simulink model "f18full_DUtrim"  (R2015a)
settings: Solver=ode45  StartTime=0.0  StopTime=10.0  RelTol=1e-3
values from neighbouring files (symbols this model uses):
  b = 37.4    [Trim_stab_f18fullDU_a.m]    (also in Trim_stab_f18fullDU_aEDIT.m)
  c = 11.52    [Trim_stab_f18fullDU_a.m]    (also in Trim_stab_f18fullDU_aEDIT.m)
  g = 32.2    [Trim_stab_f18fullDU_a.m]    (also in Trim_stab_f18fullDU_aEDIT.m)
  Ixx = 23000    [Trim_stab_f18fullDU_a.m]    (also in Trim_stab_f18fullDU_aEDIT.m)
  Ixz = - 2971    (= -2971)    [Trim_stab_f18fullDU_a.m]    (also in Trim_stab_f18fullDU_aEDIT.m)
  Iyy = 151293    [Trim_stab_f18fullDU_a.m]    (also in Trim_stab_f18fullDU_aEDIT.m)
  Izz = 169945    [Trim_stab_f18fullDU_a.m]    (also in Trim_stab_f18fullDU_aEDIT.m)
  m = 1034.5    [Trim_stab_f18fullDU_a.m]    (also in Trim_stab_f18fullDU_aEDIT.m)
  rho = 1.0660e-003    (= 0.001066)    [Trim_stab_f18fullDU_a.m]    (also in Trim_stab_f18fullDU_aEDIT.m)
  S = 400    [Trim_stab_f18fullDU_a.m]    (also in Trim_stab_f18fullDU_aEDIT.m)
  x = x_init    [Trim_stab_f18fullDU_a.m]    (also in Trim_stab_f18fullDU_aEDIT.m)
undefined symbols (not defined in the file or in its folder): CD0, CDalpha0, CDalpha1, CDalpha2, CDalpha3, CDalpha4, CDdeltastab0, CDdeltastab1, CDdeltastab2, CDdeltastab3, CLalpha0, CLalpha1, CLalpha2, CLalpha3, CLdeltastab0, CLdeltastab1, CLdeltastab2, CLdeltastab3, CMalpha0, CMalpha1, CMalpha2, CMdeltastab0, CMdeltastab1, CMdeltastab2, CMq0, CMq1, CMq2, CMq3, Cnbeta0, Cnbeta1, Cnbeta2, Cndeltaail0, Cndeltaail1, Cndeltaail2, Cndeltaail3, Cndeltarud0, Cndeltarud1, Cndeltarud2, Cndeltarud3, Cndeltarud4, Cnp0, Cnp1, Cnr0, Cnr1, CYbeta0, CYbeta1, CYbeta2, CYdeltaail0, CYdeltaail1, CYdeltaail2, CYdeltaail3, CYdeltarud0, CYdeltarud1, CYdeltarud2, CYdeltarud3
settings Model: Creator=BC  LastModifiedBy=BC
settings DataIOCC: SignalLoggingSaveFormat=ModelDataLogs
settings OptimizationCC: ExpressionDepthLimit=2147483647
settings DebuggingCC: UnderspecifiedInitializationDetection=Classic  MergeDetectMultiDrivingBlocksExec=none  SolverPrmCheckMsg=warning  FcnCallInpInsideContextMsg=EnableAllAsWarning  StateNameClashWarn=warning
settings GRTTargetCC: CombineOutputUpdateFcns=off  GRTInterface=on

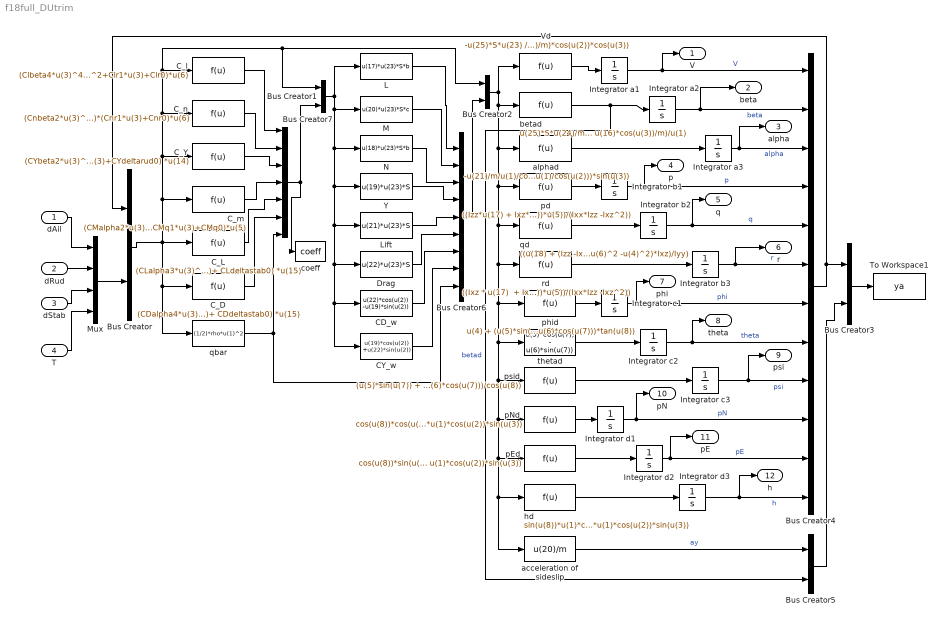
== system f18full_DUtrim ==
  dAil : Inport
  dRud : Inport  Port=2
  dStab : Inport  Port=3
  T : Inport  Port=4
  Bus Creator{,1..3,5} (5 alike) : BusCreator  Inputs=2
  Bus Creator4 : BusCreator  Inputs=12
  Bus Creator6 : BusCreator  Inputs=9
  Bus Creator7 : BusCreator  Inputs=7
  CD_w : Fcn  Expr=u(22)*cos(u(2)) -u(19)*sin(u(2))
  CY_w : Fcn  Expr=u(19)*cos(u(2)) +u(22)*sin(u(2))
  C_D : Fcn  Expr=(CDalpha4*u(3)^4+CDalpha3*u(3)^3+CDalpha2*u(3)^2+CDalpha1*u(3)+CDalpha0)*cos(u(2))+CD0 +(CDdeltastab3*u(3)^3+ CDdeltastab2*u(3)^2+ CDdeltastab1*u(3)+ CDdeltastab0) *u(15)
  C_L : Fcn  Expr=(CLalpha3*u(3)^3+CLalpha2*u(3)^2+CLalpha1*u(3)+CLalpha0)*cos(2*u(2)/3)+(CLdeltastab3*u(3)^3+ CLdeltastab2*u(3)^2+ CLdeltastab1*u(3)+ CLdeltastab0) *u(15)
  C_Y : Fcn  Expr=(CYbeta2*u(3)^2+CYbeta1*u(3)+CYbeta0)*u(2)+(CYdeltaail3*u(3)^3+CYdeltaail2*u(3)^2+CYdeltaail1*u(3)+CYdeltaail0)*u(13)+(CYdeltarud3*u(3)^3+CYdeltarud2*u(3)^2+CYdeltarud1*u(3)+CYdeltarud0) *u(14)
  C_l : Fcn  Expr=(Clbeta4*u(3)^4+Clbeta3*u(3)^3+Clbeta2*u(3)^2+Clbeta1*u(3)+Clbeta0)*u(2)+(Cldeltaail3*u(3)^3+Cldeltaail2*u(3)^2+Cldeltaail1*u(3)+Cldeltaail0)*u(13)+(Cldeltarud3*u(3)^3+Cldeltarud2*u(3)^2+Cldeltarud1*u(3)+Cldeltarud0)*u(14)+(b/(2*u(1)))*(Clp1*u(3)+Clp0)*u(4)+(b/(2*u(1)))*(Clr2*u(3)^2+Clr1*u(3)+Clr0)*u(6)
  C_m : Fcn  Expr=(CMalpha2*u(3)^2+CMalpha1*u(3)+CMalpha0)+(CMdeltastab2*u(3)^2+CMdeltastab1*u(3)+CMdeltastab0)*u(15)+(c/(2*u(1)))*(CMq3*u(3)^3+CMq2*u(3)^2+CMq1*u(3)+CMq0)*u(5)
  C_n : Fcn  Expr=(Cnbeta2*u(3)^2+Cnbeta1*u(3)+Cnbeta0)*u(2)+(Cndeltarud4*u(3)^4+Cndeltarud3*u(3)^3+Cndeltarud2*u(3)^2+Cndeltarud1*u(3)+Cndeltarud0)*u(14)+(Cndeltaail3*u(3)^3+Cndeltaail2*u(3)^2+Cndeltaail1*u(3)+Cndeltaail0)*u(13)+(b/(2*u(1)))*(Cnp1*u(3)+Cnp0)*u(4)+(b/(2*u(1)))*(Cnr1*u(3)+Cnr0)*u(6)
  Drag : Fcn  Expr=u(22)*u(23)*S
  Integrator a1 : Integrator  InitialCondition=x(1)
  Integrator a2 : Integrator  InitialCondition=x(2)
  Integrator a3 : Integrator  InitialCondition=x(3)
  Integrator b1 : Integrator  InitialCondition=x(4)
  Integrator b2 : Integrator  InitialCondition=x(5)
  Integrator b3 : Integrator  InitialCondition=x(6)
  Integrator c1 : Integrator  InitialCondition=x(7)
  Integrator c2 : Integrator  InitialCondition=x(8)
  Integrator c3 : Integrator  InitialCondition=x(9)
  Integrator d1 : Integrator  InitialCondition=x(10)
  Integrator d2 : Integrator  InitialCondition=x(11)
  Integrator d3 : Integrator  InitialCondition=x(12)
  L : Fcn  Expr=u(17)*u(23)*S*b
  Lift : Fcn  Expr=u(21)*u(23)*S
  M : Fcn  Expr=u(20)*u(23)*S*c
  Mux : Mux
  N : Fcn  Expr=u(18)*u(23)*S*b
  To Workspace1 : ToWorkspace  VariableName=ya  SampleTime=-1
  Vd : Fcn  Expr=-u(25)*S*u(23) /m + g*(cos(u(7))*cos(u(8))*sin(u(3))*cos(u(2)) +sin(u(7))*cos(u(8))*sin(u(2)) -sin(u(8))*cos(u(3))*cos(u(2)))+ (u(16)/m)*cos(u(2))*cos(u(3))
  Y : Fcn  Expr=u(19)*u(23)*S
  acceleration of sideslip : Fcn  Expr=u(20)/m
  alphad : Fcn  Expr=-u(21)/m/u(1)/cos(u(2)) + u(5) - tan(u(2))*(u(4)*cos(u(3))+u(6)*sin(u(3)))+ g*(cos(u(7))*cos(u(8))*cos(u(3)) + sin(u(8))*sin(u(3)))/u(1)/cos(u(2))-(u(16)/m/u(1)/cos(u(2)))*sin(u(3))
  betad : Fcn  Expr=u(25)*S*u(24)/m/u(1) + u(4)*sin(u(3))-u(6)*cos(u(3)) +g*cos(u(8))*sin(u(7))*cos(u(2))/u(1) + sin(u(2))*(g*cos(u(3))*sin(u(8))- g*sin(u(3))*cos(u(7))*cos(u(8))+ u(16)*cos(u(3))/m)/u(1)
  coeff : ToWorkspace  VariableName=coeff  SampleTime=-1
  hd : Fcn  Expr=sin(u(8))*u(1)*cos(u(2))*cos(u(3))-sin(u(7))*cos(u(8))*u(1)*sin(u(2))-cos(u(7))*cos(u(8))*u(1)*cos(u(2))*sin(u(3))
  pEd : Fcn  Expr=cos(u(8))*sin(u(9))* u(1)*cos(u(2))*cos(u(3)) +(sin(u(7))*sin(u(8))*sin(u(9))+cos(u(7))*cos(u(9)))* u(1)*sin(u(2)) +(cos(u(7))*sin(u(8))*sin(u(9))-sin(u(7))*cos(u(9)))* u(1)*cos(u(2))*sin(u(3))
  pNd : Fcn  Expr=cos(u(8))*cos(u(9))*u(1)*cos(u(2))*cos(u(3))+(sin(u(7))*sin(u(8))*cos(u(9))-cos(u(7))*sin(u(9)))*u(1)*sin(u(2))+(cos(u(7))*sin(u(8))*cos(u(9))+sin(u(7))*sin(u(9)))*u(1)*cos(u(2))*sin(u(3))
  pd : Fcn  Expr=((Izz*u(17) + Ixz*u(19) - (Ixz*(Iyy-Ixx-Izz)*u(4) +(Ixz^2 + Izz*(Izz - Iyy))*u(6))*u(5))/(Ixx*Izz -Ixz^2))
  phid : Fcn  Expr=u(4) + (u(5)*sin(u(7)) + u(6)*cos(u(7)))*tan(u(8))
  psid : Fcn  Expr=(u(5)*sin(u(7)) + u(6)*cos(u(7)))/cos(u(8))
  qbar : Fcn  Expr=(1/2)*rho*u(1)^2
  qd : Fcn  Expr=((u(18) + (Izz -Ixx)*u(4)*u(6) + (u(6)^2 -u(4)^2)*Ixz)/Iyy)
  rd : Fcn  Expr="((Ixz * u(17)  + Ixx * u(19) + (Ixz * (Iyy - Ixx -Izz) *u(6) +(Ixz^2 + Ixx*(Ixx - Iyy))*u(4))*u(5))/(Ixx*Izz -Ixz^2))"
  thetad : Fcn  Expr=u(5)*cos(u(7)) - u(6)*sin(u(7))
  V : Outport
  beta : Outport  Port=2
  alpha : Outport  Port=3
  p : Outport  Port=4
  q : Outport  Port=5
  r : Outport  Port=6
  phi : Outport  Port=7
  theta : Outport  Port=8
  psi : Outport  Port=9
  pN : Outport  Port=10
  pE : Outport  Port=11
  h : Outport  Port=12
  wires:
  pd/1 -> Integrator b1/1
  phid/1 -> Integrator c1/1
  alphad/1 -> Integrator a3/1
  thetad/1 -> Integrator c2/1
  qd/1 -> Integrator b2/1
  Bus Creator4/1 -> Bus Creator3/1, Bus Creator/1
  psid/1 -> Integrator c3/1
  hd/1 -> Integrator d3/1
  pEd/1 -> Integrator d2/1
  rd/1 -> Integrator b3/1
  pNd/1 -> Integrator d1/1
  Integrator b2/1 -> Bus Creator4/5, q/1  "q"
  Bus Creator/1 -> C_L/1, C_D/1, qbar/1, Bus Creator1/1, Bus Creator2/1, C_l/1, C_n/1, C_Y/1, C_m/1
  Bus Creator2/1 -> Vd/1, betad/1, alphad/1, qd/1, thetad/1, psid/1, pNd/1, pEd/1, hd/1, acceleration of sideslip/1, phid/1, rd/1, pd/1
  Integrator c1/1 -> Bus Creator4/7, phi/1  "phi"
  Integrator d2/1 -> Bus Creator4/11, pE/1  "pE"
  Vd/1 -> Integrator a1/1
  betad/1 -> Integrator a2/1, Bus Creator5/2  "betad"
  Integrator d3/1 -> Bus Creator4/12, h/1  "h"
  Bus Creator1/1 -> L/1, M/1, N/1, Y/1, Lift/1, Drag/1, CD_w/1, CY_w/1
  Bus Creator7/1 -> Bus Creator1/2, coeff/1
  C_m/1 -> Bus Creator7/4
  C_l/1 -> Bus Creator7/1
  Integrator b1/1 -> Bus Creator4/4, p/1  "p"
  C_n/1 -> Bus Creator7/2
  Integrator a3/1 -> Bus Creator4/3, alpha/1  "alpha"
  qbar/1 -> Bus Creator7/7, Bus Creator6/9
  Integrator c3/1 -> Bus Creator4/9, psi/1  "psi"
  Bus Creator6/1 -> Bus Creator2/2
  Integrator a2/1 -> Bus Creator4/2, beta/1  "beta"
  Integrator a1/1 -> Bus Creator4/1, V/1  "V"
  Integrator b3/1 -> Bus Creator4/6, r/1  "r"
  C_Y/1 -> Bus Creator7/3
  Mux/1 -> Bus Creator/2
  Integrator c2/1 -> Bus Creator4/8, theta/1  "theta"
  Integrator d1/1 -> Bus Creator4/10, pN/1  "pN"
  L/1 -> Bus Creator6/1
  M/1 -> Bus Creator6/2
  N/1 -> Bus Creator6/3
  Y/1 -> Bus Creator6/4
  Lift/1 -> Bus Creator6/5
  Drag/1 -> Bus Creator6/6
  CD_w/1 -> Bus Creator6/7
  CY_w/1 -> Bus Creator6/8
  C_L/1 -> Bus Creator7/5
  C_D/1 -> Bus Creator7/6
  acceleration of sideslip/1 -> Bus Creator5/1  "ay"
  Bus Creator5/1 -> Bus Creator3/2
  Bus Creator3/1 -> To Workspace1/1
  dAil/1 -> Mux/1
  dRud/1 -> Mux/2
  T/1 -> Mux/4
  dStab/1 -> Mux/3
